simulink model "launcher_position"  (R2018b)
settings: Solver=VariableStepAuto  StartTime=0.0  StopTime=10.0  RelTol=1e-3
settings Model: Creator=12819  LastModifiedBy=12819

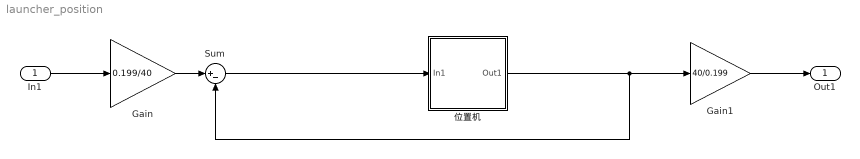
== system launcher_position ==
  In1 : Inport
  Gain : Gain  Gain=0.199/40
  Gain1 : Gain  Gain=40/0.199
  Sum : Sum  Inputs=|+-
  位置机 : Subsystem
  Out1 : Outport
  wires:
  Sum/1 -> 位置机/1(In1)
  Gain/1 -> Sum/1
  位置机/1(Out1) -> Sum/2, Gain1/1
  In1/1 -> Gain/1
  Gain1/1 -> Out1/1

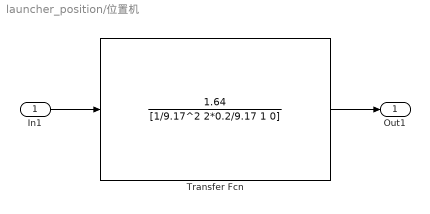
== system launcher_position/位置机 ==
  In1 : Inport
  Transfer Fcn : TransferFcn  Numerator=[1.64]  Denominator=[1/9.17^2 2*0.2/9.17 1 0]
  Out1 : Outport
  wires:
  Transfer Fcn/1 -> Out1/1
  In1/1 -> Transfer Fcn/1
